simulink model "sampleModel1860"  (R2023a)
settings: Solver=VariableStepAuto  StartTime=0.0  StopTime=10.0  RelTol=1e-3
libraries: simulink x3, hdlsllib x3
settings Model: Creator=user1  LastModifiedBy=user1

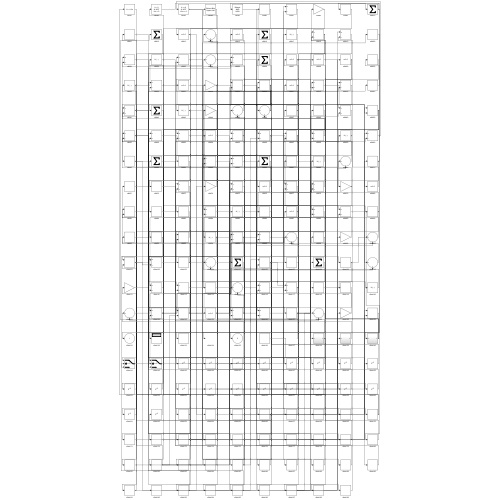
[thumbnail: Simulink's stored preview of the top-level diagram]
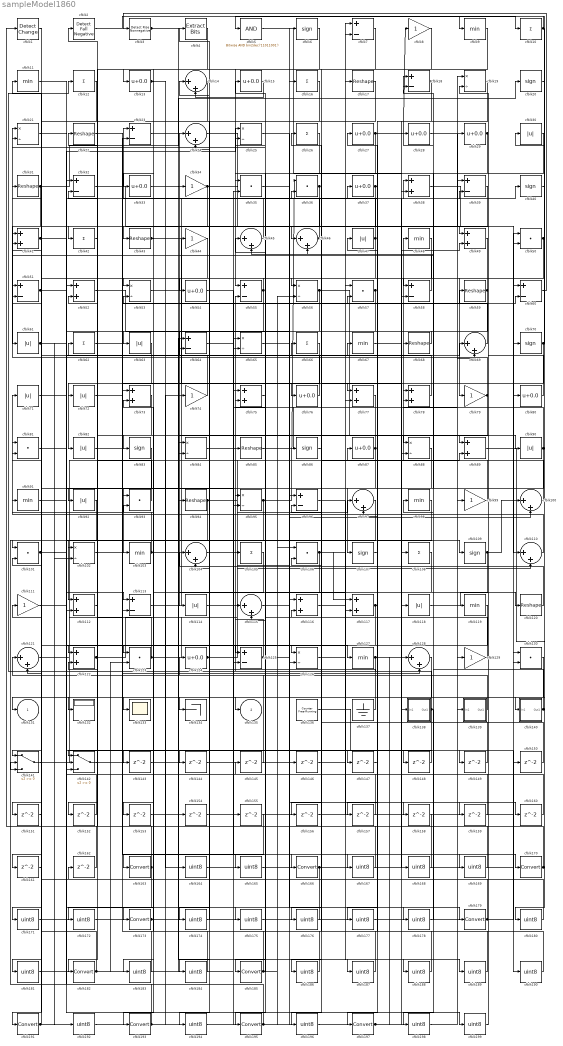
== system sampleModel1860 ==
  cfblk1 : simulink/Logic and Bit Operations/Detect Change  vinit=0  OutDataTypeStr=boolean
      settings: LibrarySourceBlock=|
      | hdlsllib/Logic and Bit
      | Operations/Detect
      | Change
  cfblk{10,12,16,26,42,62,66,105,108} (9 alike) : Sum  Inputs=+
  cfblk{14,24,45..46,69,97,100,104,110,115,121,128} (12 alike) : Sum  Inputs=|++
  cfblk{35..36,50,57,81,93,101,106,123,130} (10 alike) : DotProduct  OutDataTypeStr=Inherit: Inherit via internal rule
  cfblk{19,21,25,53,56,65,84,88,95,102,126} (11 alike) : Product  Inputs=*/  RndMeth=Zero  SaturateOnIntegerOverflow=on
  cfblk{9,11,48,67,91,98,103,119,127} (9 alike) : MinMax
  cfblk{6,20,40,70,83,86,107,109} (8 alike) : Signum
  cfblk{8,34,44,74,79,99,111,129} (8 alike) : Gain
  cfblk{38,41,49,52,73,75,77..78,89,112,116..117,122} (13 alike) : Sum
  cfblk{7,18,23,32,39,51,55,58,60,64,96,113,125} (13 alike) : Sum  Inputs=+-
  cfblk{30,47,61,63,71..72,82,90,92,114,118} (11 alike) : Abs  SaturateOnIntegerOverflow=off
  cfblk{17,22,31,43,59,68,85,94,120} (9 alike) : Reshape
  cfblk{13,15,27..29,33,37,54,76,80,87,124} (12 alike) : Bias  Bias=0.0  SaturateOnIntegerOverflow=off
  cfblk132 : Display
  cfblk133 : Scope
  cfblk134 : Terminator
  cfblk136 : hdlsllib/Sources/Counter Free-Running  NumBits=16  tsamp=-1
  cfblk137 : Ground
  cfblk138 : Subsystem
      settings: LibrarySourceBlock=|
      | hdlsllib/Ports &
      | Subsystems/Subsystem
  cfblk139 : Subsystem
      settings: LibrarySourceBlock=|
      | hdlsllib/Ports &
      | Subsystems/Subsystem
  cfblk140 : Subsystem
      settings: LibrarySourceBlock=|
      | hdlsllib/Ports &
      | Subsystems/Subsystem
  cfblk141 : Switch  SaturateOnIntegerOverflow=off  InputSameDT=off
  cfblk142 : Switch  SaturateOnIntegerOverflow=off  InputSameDT=off
  cfblk{143..162} (20 alike) : Delay  SampleTime=1
  cfblk{163,166,170,173,179,182,185,191,193,195,197} (11 alike) : DataTypeConversion  SaturateOnIntegerOverflow=off  RndMeth=Floor
  cfblk{164..165,167..169,171..172,174..178,180..181,183..184,186..190,192,194,196,198..199} (26 alike) : DataTypeConversion  OutDataTypeStr=uint8  SaturateOnIntegerOverflow=off  RndMeth=Floor
  cfblk2 : hdlsllib/Logic and Bit Operations/Detect Fall Negative  vinit=0  OutDataTypeStr=boolean
  cfblk3 : hdlsllib/Logic and Bit Operations/Detect Rise Nonnegative  vinit=0  OutDataTypeStr=boolean
  cfblk4 : simulink/Logic and Bit Operations/Extract Bits  bitsToExtract=Upper half  numBits=8  bitIdxRange=[0 7]  outScalingMode=Preserve fixed-point scaling
      settings: LibrarySourceBlock=|
      | hdlsllib/Logic and Bit
      | Operations/Extract Bits
  cfblk5 : simulink/Logic and Bit Operations/Bitwise Operator  logicop=AND  UseBitMask=on  BitMask=bin2dec('11011001')  BitMaskRealWorld=Stored Integer
      settings: LibrarySourceBlock=|
      | hdlsllib/Logic and Bit
      | Operations/Bitwise
      | Operator
  cfblk131 : Outport  VectorParamsAs1DForOutWhenUnconnected=off
  cfblk135 : Outport  Port=2  VectorParamsAs1DForOutWhenUnconnected=off
  wires:
  cfblk13/1 -> cfblk33/1, cfblk164/1
  cfblk64/1 -> cfblk170/1
  cfblk6/1 -> cfblk55/1
  cfblk113/1 -> cfblk38/1
  cfblk66/1 -> cfblk82/1
  cfblk127/1 -> cfblk12/1, cfblk60/2, cfblk49/2, cfblk39/2
  cfblk89/1 -> cfblk131/1
  cfblk141/1 -> cfblk48/1
  cfblk22/1 -> cfblk166/1
  cfblk95/1 -> cfblk36/1, cfblk142/3
  cfblk30/1 -> cfblk107/1
  cfblk24/1 -> cfblk49/1
  cfblk116/1 -> cfblk7/1
  cfblk40/1 -> cfblk5/1
  cfblk56/1 -> cfblk89/1, cfblk115/2
  cfblk112/1 -> cfblk2/1
  cfblk9/1 -> cfblk42/1
  cfblk90/1 -> cfblk68/1, cfblk181/1
  cfblk49/1 -> cfblk132/1
  cfblk84/1 -> cfblk55/2
  cfblk5/1 -> cfblk38/2
  cfblk60/1 -> cfblk3/1
  cfblk68/1 -> cfblk63/1
  cfblk3/1 -> cfblk117/2, cfblk165/1
  cfblk57/1 -> cfblk114/1, cfblk142/2
  cfblk10/1 -> cfblk9/1, cfblk180/1
  cfblk61/1 -> cfblk41/2, cfblk25/1, cfblk192/1
  cfblk94/1 -> cfblk89/2, cfblk141/3
  cfblk16/1 -> cfblk191/1
  cfblk28/1 -> cfblk50/2
  cfblk50/1 -> cfblk79/1, cfblk54/1, cfblk151/1
  cfblk108/1 -> cfblk195/1
  cfblk124/1 -> cfblk97/1, cfblk78/2
  cfblk105/1 -> cfblk193/1
  cfblk93/1 -> cfblk52/2
  cfblk73/1 -> cfblk182/1
  cfblk83/1 -> cfblk103/1
  cfblk109/1 -> cfblk100/1, cfblk186/1
  cfblk8/1 -> cfblk13/1
  cfblk103/1 -> cfblk87/1, cfblk31/1
  cfblk106/1 -> cfblk117/1, cfblk126/2, cfblk169/1
  cfblk118/1 -> cfblk120/1
  cfblk55/1 -> cfblk53/1, cfblk72/1
  cfblk76/1 -> cfblk24/1
  cfblk78/1 -> cfblk45/1
  cfblk51/1 -> cfblk109/1, cfblk199/1
  cfblk19/1 -> cfblk197/1
  cfblk2/1 -> cfblk10/1
  cfblk18/1 -> cfblk77/1, cfblk58/2
  cfblk117/1 -> cfblk37/1, cfblk184/1
  cfblk75/1 -> cfblk185/1
  cfblk36/1 -> cfblk141/1, cfblk94/1, cfblk134/1
  cfblk138/1(Out1) -> cfblk85/1, cfblk196/1, cfblk198/1
  cfblk77/1 -> cfblk83/1
  cfblk79/1 -> cfblk21/1, cfblk135/1
  cfblk31/1 -> cfblk61/1, cfblk20/1
  cfblk46/1 -> cfblk34/1, cfblk25/2
  cfblk62/1 -> cfblk76/1
  cfblk54/1 -> cfblk88/1
  cfblk52/1 -> cfblk116/1
  cfblk20/1 -> cfblk140/1(In1)
  cfblk27/1 -> cfblk8/1, cfblk126/1, cfblk159/1
  cfblk53/1 -> cfblk88/2
  cfblk65/1 -> cfblk179/1
  cfblk129/1 -> cfblk21/2
  cfblk47/1 -> cfblk23/1, cfblk84/2
  cfblk38/1 -> cfblk80/1
  cfblk92/1 -> cfblk112/1
  cfblk102/1 -> cfblk128/2
  cfblk74/1 -> cfblk51/1
  cfblk137/1 -> cfblk14/1
  cfblk80/1 -> cfblk53/2
  cfblk29/1 -> cfblk58/1, cfblk35/1
  cfblk140/1(Out1) -> cfblk45/2, cfblk104/1, cfblk44/1
  cfblk123/1 -> cfblk17/1, cfblk115/1, cfblk32/2
  cfblk121/1 -> cfblk23/2
  cfblk14/1 -> cfblk43/1
  cfblk99/1 -> cfblk26/1
  cfblk11/1 -> cfblk113/1
  cfblk33/1 -> cfblk90/1
  cfblk32/1 -> cfblk110/1
  cfblk69/1 -> cfblk18/1
  cfblk88/1 -> cfblk133/1
  cfblk26/1 -> cfblk125/1
  cfblk58/1 -> cfblk41/1
  cfblk110/1 -> cfblk71/1
  cfblk100/1 -> cfblk47/1
  cfblk142/1 -> cfblk6/1
  cfblk63/1 -> cfblk122/1
  cfblk120/1 -> cfblk36/2
  cfblk34/1 -> cfblk138/1(In1), cfblk143/1
  cfblk125/1 -> cfblk95/1, cfblk100/2
  cfblk43/1 -> cfblk125/2, cfblk123/1
  cfblk7/1 -> cfblk46/1
  cfblk104/1 -> cfblk57/1
  cfblk48/1 -> cfblk113/2
  cfblk59/1 -> cfblk56/1, cfblk104/2
  cfblk21/1 -> cfblk95/2
  cfblk139/1(Out1) -> cfblk124/1
  cfblk15/1 -> cfblk14/2
  cfblk70/1 -> cfblk30/1, cfblk156/1
  cfblk85/1 -> cfblk39/1
  cfblk1/1 -> cfblk101/1
  cfblk101/1 -> cfblk81/1, cfblk40/1, cfblk102/2
  cfblk122/1 -> cfblk78/1, cfblk86/1
  cfblk114/1 -> cfblk110/2
  cfblk82/1 -> cfblk59/1
  cfblk41/1 -> cfblk127/1, cfblk149/1
  cfblk4/1 -> cfblk173/1
  cfblk12/1 -> cfblk112/2
  cfblk44/1 -> cfblk102/1
  cfblk87/1 -> cfblk84/1, cfblk194/1
  cfblk37/1 -> cfblk97/2, cfblk92/1
  cfblk130/1 -> cfblk163/1
  cfblk45/1 -> cfblk24/2
  cfblk81/1 -> cfblk69/1
  cfblk39/1 -> cfblk144/1
  cfblk144/1 -> cfblk77/2
  cfblk145/1 -> cfblk121/1
  cfblk115/1 -> cfblk146/1
  cfblk146/1 -> cfblk116/2
  cfblk71/1 -> cfblk147/1
  cfblk147/1 -> cfblk57/2
  cfblk72/1 -> cfblk148/1
  cfblk148/1 -> cfblk142/1
  cfblk149/1 -> cfblk46/2
  cfblk150/1 -> cfblk106/2
  cfblk151/1 -> cfblk51/2
  cfblk42/1 -> cfblk152/1
  cfblk152/1 -> cfblk52/1
  cfblk97/1 -> cfblk153/1
  cfblk153/1 -> cfblk7/2
  cfblk154/1 -> cfblk69/2
  cfblk156/1 -> cfblk60/1
  cfblk107/1 -> cfblk157/1
  cfblk157/1 -> cfblk122/2
  cfblk35/1 -> cfblk158/1
  cfblk158/1 -> cfblk1/1
  cfblk159/1 -> cfblk93/2
  cfblk126/1 -> cfblk160/1
  cfblk160/1 -> cfblk18/2
  cfblk119/1 -> cfblk161/1
  cfblk161/1 -> cfblk81/2
  cfblk162/1 -> cfblk101/2
  cfblk163/1 -> cfblk62/1, cfblk172/1
  cfblk164/1 -> cfblk130/1
  cfblk165/1 -> cfblk130/2
  cfblk166/1 -> cfblk162/1, cfblk129/1
  cfblk25/1 -> cfblk167/1
  cfblk167/1 -> cfblk22/1
  cfblk67/1 -> cfblk168/1
  cfblk168/1 -> cfblk121/2
  cfblk169/1 -> cfblk67/1
  cfblk170/1 -> cfblk145/1, cfblk66/1
  cfblk128/1 -> cfblk171/1
  cfblk171/1 -> cfblk64/1
  cfblk172/1 -> cfblk64/2
  cfblk173/1 -> cfblk155/1, cfblk70/1, cfblk139/1(In1)
  cfblk17/1 -> cfblk174/1
  cfblk174/1 -> cfblk4/1
  cfblk91/1 -> cfblk175/1
  cfblk175/1 -> cfblk29/1
  cfblk86/1 -> cfblk176/1
  cfblk176/1 -> cfblk91/1
  cfblk98/1 -> cfblk177/1
  cfblk177/1 -> cfblk50/1
  cfblk111/1 -> cfblk178/1
  cfblk178/1 -> cfblk98/1
  cfblk179/1 -> cfblk150/1, cfblk28/1
  cfblk180/1 -> cfblk65/1
  cfblk181/1 -> cfblk65/2
  cfblk182/1 -> cfblk154/1, cfblk35/2, cfblk123/2, cfblk11/1
  cfblk155/1 -> cfblk183/1
  cfblk183/1 -> cfblk73/1
  cfblk184/1 -> cfblk73/2
  cfblk185/1 -> cfblk15/1, cfblk56/2, cfblk93/1
  cfblk186/1 -> cfblk75/1
  cfblk143/1 -> cfblk187/1
  cfblk187/1 -> cfblk75/2
  cfblk96/1 -> cfblk188/1
  cfblk188/1 -> cfblk27/1
  cfblk23/1 -> cfblk189/1
  cfblk189/1 -> cfblk96/1
  cfblk136/1 -> cfblk190/1
  cfblk190/1 -> cfblk96/2
  cfblk191/1 -> cfblk118/1, cfblk111/1
  cfblk192/1 -> cfblk16/1
  cfblk193/1 -> cfblk141/2, cfblk74/1
  cfblk194/1 -> cfblk105/1
  cfblk195/1 -> cfblk32/1, cfblk106/1
  cfblk196/1 -> cfblk108/1
  cfblk197/1 -> cfblk119/1, cfblk99/1, cfblk128/1
  cfblk198/1 -> cfblk19/1
  cfblk199/1 -> cfblk19/2

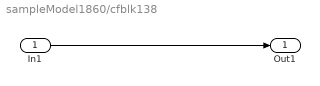
== system sampleModel1860/cfblk138 ==
  In1 : Inport
  Out1 : Outport
  wires:
  In1/1 -> Out1/1

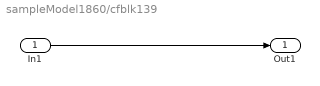
== system sampleModel1860/cfblk139 ==
  In1 : Inport
  Out1 : Outport
  wires:
  In1/1 -> Out1/1

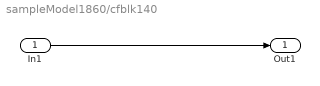
== system sampleModel1860/cfblk140 ==
  In1 : Inport
  Out1 : Outport
  wires:
  In1/1 -> Out1/1
